simulink model "Telemetry_Test"  (Simulink 7.7)
settings: Solver=ode4  StartTime=0.0  StopTime=inf  FixedStep=sample_time_Vicon  RelTol=1e-3
InitFcn:
  | sample_time_Vicon = 0.004;
  | sample_time=0.02;
  | DeltaT = sample_time;
  | H0 = -0.36;
  | Kl = 1;
  | Omega_r =1.1; %1.3
settings Model: Creator=ttcl3  LastModifiedBy=Vicon
settings SolverCC: MaxConsecutiveMinStep=auto
settings OptimizationCC: EfficientMapNaN2IntZero=off
settings DebuggingCC: MultiTaskRateTransMsg=warning
settings HardwareCC: TargetIntDivRoundTo=Zero  TargetEndianess=LittleEndian  TargetHWDeviceType=MATLAB Host  ProdEqTarget=off
settings SFSimCC: SimParseCustomCode=off
settings CodeAppCC: MaxIdLength=128

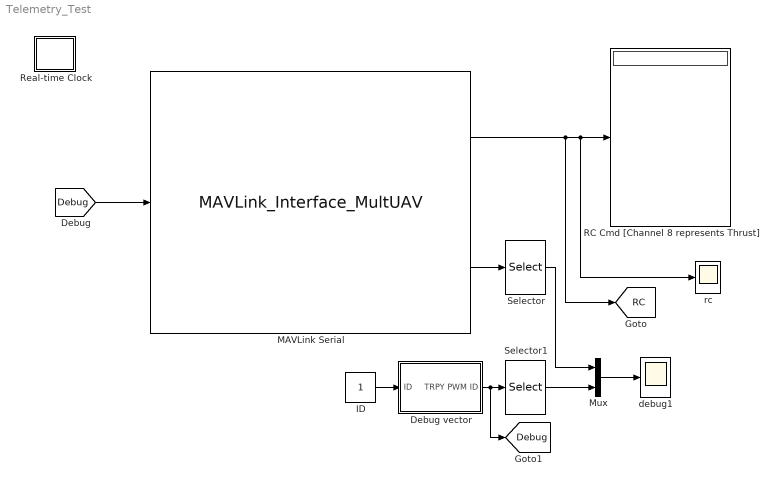
== system Telemetry_Test ==
  Debug vector : Subsystem
  ID : Constant
  MAVLink Serial : S-Function  FunctionName=MAVLink_Interface_MultUAV  Parameters=COM_Port,Baud_Rate,MSG_INPUT,MSG_OUTPUT  EnableBusSupport=off  mask{COM_Port='COM7', Baud_Rate=57600, ATTITUDE_OUT=on, RC_SCALED=on, Quad_1=off, Quad_2=off, Quad_3=off, Quad_4=off, Quad_5=off, Quad_6=off, Quad_7=on, Quad_8=off, Quad_9=off, Quad_10=off, Quad_11=off, Quad_12=off, Quad_13=off, Quad_14=off, Quad_15=off, Quad_16=off, Quad_17=off, Quad_18=off, Quad_19=off, Quad_20=off, Quad_21=off, Quad_22=off, Quad_23=off, Quad_24=off, Quad_25=off, Quad_26=off, Quad_27=off, Quad_28=off, Quad_29=off, Quad_30=off}
      mask prompts: COM_Port "COM Port"; Baud_Rate "Baud Rate"; ATTITUDE_OUT "ATTITUDE"; RC_SCALED "RC CHANNELS SCALED"; Quad_1 "Quad No 1"; Quad_2 "Quad No 2"; Quad_3 "Quad No 3"; Quad_4 "Quad No 4"; Quad_5 "Quad No 5"; Quad_6 "Quad No 6"; Quad_7 "Quad No 7"; Quad_8 "Quad No 8"; Quad_9 "Quad No 9"; Quad_10 "Quad No 10"; Quad_11 "Quad No 11"; Quad_12 "Quad No 12"; Quad_13 "Quad No 13"; Quad_14 "Quad No 14"; Quad_15 "Quad No 15"; Quad_16 "Quad No 16"; Quad_17 "Quad No 17"; Quad_18 "Quad No 18"; Quad_19 "Quad No 19"; Quad_20 "Quad No 20"; Quad_21 "Quad No 21"; Quad_22 "Quad No 22"; Quad_23 "Quad No 23"; Quad_24 "Quad No 24"; Quad_25 "Quad No 25"; Quad_26 "Quad No 26"; Quad_27 "Quad No 27"; Quad_28 "Quad No 28"; Quad_29 "Quad No 29"; Quad_30 "Quad No 30"
      mask init:
      | MSG_ID_NUM_INPUT = [uint8(196) uint8(197) uint8(198) uint8(199) uint8(200) uint8(201) uint8(202) uint8(203) uint8(204) uint8(205)
      |                     uint8(206) uint8(207) uint8(208) uint8(209) uint8(210) uint8(211) uint8(212) uint8(213) uint8(214) uint8(215)
      |                     uint8(216) uint8(217) uint8(218) uint8(219) uint8(220) uint8(221) uint8(222) uint8(223) uint8(224) uint8(225)];
      | MSG_ID_NAME_INPUT = [Quad_1 Quad_2 Quad_3 Quad_4 Quad_5 Quad_6 Quad_7 Quad_8 Quad_9 Quad_10
      |                      Quad_11 Quad_12 Quad_13 Quad_14 Quad_15 Quad_16 Quad_17 Quad_18 Quad_19 Quad_20
      |                      Quad_21 Quad_22 Quad_23 Quad_24 Quad_25 Quad_26 Quad_27 Quad_28 Quad_29 Quad_30];
      | 
      | MSG_ID_NUM_OUTPUT = [uint8(34) uint8(30)];
      | MSG_ID_NAME_OUTPUT = [RC_SCALED ATTITUDE_OUT ];
      | 
      | idx_input = find(MSG_ID_NAME_INPUT);
      | MSG_INPUT = MSG_ID_NUM_INPUT(idx_input);
      | 
      | idx_output = find(MSG_ID_NAME_OUTPUT);
      | MSG_OUTPUT = MSG_ID_NUM_OUTPUT(idx_output);
      mask TabNameString: Setting,Setting,Output Message,Output Message,Input Message,Input Message,Input Message,Input Message,Input Message,Input Message,Input Message,Input Message,Input Message,Input Message,Input Message,Input Message,Input Message,Input Message,Input Message,Input Message,Input Message,Input Message,Input Message,Input Message,Input Message,Input Message,Input Message,Input Message,Input Message,Input Message,Input Message,Input Message,Input Message,Input Message
      mask Display:
      | % Block image
      | image(imread('10-inch Quad Heat Map.png'));
      | 
      | %Label block
      | fprintf('MAVLink Serial\n%s\n%dbps', COM_Port,  Baud_Rate)
      | 
      | 
      | %Label input ports
      | 
      | in = 1;
      | if (Quad_1 == 1)
      |     port_label('input', in, 'Quad 1');
      |     in = in + 1;
      | end
      | if (Quad_2 == 1)
      |     port_label('input', in, 'Quad 2');
      |     in = in + 1;
      | end
      | 
      | if (Quad_3 == 1)
      |     port_label('input', in, 'Quad 3');
      |     in = in + 1;
      | end
      | 
      | if (Quad_4 == 1)
      |     port_label('input', in, 'Quad 4');
      |     in = in + 1;
      | end
      | 
      | if (Quad_5 == 1)
      |     port_label('input', in, 'Quad 5');
      |     in = in + 1;
      | end
      | 
      | if (Quad_6 == 1)
      |     port_label('input', in, 'Quad 6');
      |     in = in + 1;
      | end
      | 
      | if (Quad_7 == 1)
      |     port_label('input', in, 'Quad 7');
      |     in = in + 1;
      | end
      | 
      | if (Quad_8 == 1)
      |     port_label('input', in, 'Quad 8');
      |     in = in + 1;
      | end
      | 
      | if (Quad_9 == 1)
      |     port_label('input', in, 'Quad 9');
      |     in = in + 1;
      | end
      | 
      | if (Quad_10 == 1)
      |     port_label('input', in, 'Quad 10');
      |     in = in + 1;
      | end
      | 
      | if (Quad_11 == 1)
      |     port_label('input', in, 'Quad 11');
      |     in = in + 1;
      | end
      | 
      | if (Quad_12 == 1)
      |     port_label('input', in, 'Quad 12');
      |     in = in + 1;
      | end
      | 
      | if (Quad_13 == 1)
      |     port_label('input', in, 'Quad 13');
      |     in = in + 1;
      | end
      | 
      | if (Quad_14 == 1)
      |     port_label('input', in, 'Quad 14');
      |     in = in + 1;
      | end
      | 
      | if (Quad_15 == 1)
      |     port_label('input', in, 'Quad 15');
      |     in = in + 1;
      | end
      | 
      | if (Quad_16 == 1)
      |     port_label('input', in, 'Quad 16');
      |     in = in + 1;
      | end
      | 
      | if (Quad_17 == 1)
      |     port_label('input', in, 'Quad 17');
      |     in = in + 1;
      | end
      | 
      | if (Quad_18 == 1)
      |     port_label('input', in, 'Quad 18');
      |     in = in + 1;
      | end
      | 
      | 
      | if (Quad_19 == 1)
      |     port_label('input', in, 'Quad 19');
      |     in = in + 1;
      | end
      | 
      | if (Quad_20 == 1)
      |     port_label('input', in, 'Quad 20');
      |     in = in + 1;
      | end
      | 
      | if (Quad_21 == 1)
      |     port_label('input', in, 'Quad 21');
      |     in = in + 1;
      | end
      | 
      | if (Quad_22 == 1)
      |     port_label('input', in, 'Quad 22');
      |     in = in + 1;
      | end
      | 
      | if (Quad_23 == 1)
      |     port_label('input', in, 'Quad 23');
      |     in = in + 1;
      | end
      | 
      | if (Quad_24 == 1)
      |     port_label('input', in, 'Quad 24');
      |     in = in + 1;
      | end
      | 
      | if (Quad_25 == 1)
      |     port_label('input', in, 'Quad 25');
      |     in = in + 1;
      | end
      | 
      | if (Quad_26 == 1)
      |     port_label('input', in, 'Quad 26');
      |     in = in + 1;
      | end
      | 
      | if (Quad_27 == 1)
      |     port_label('input', in, 'Quad 27');
      |     in = in + 1;
      | end
      | 
      | if (Quad_28 == 1)
      |     port_label('input', in, 'Quad 28');
      |     in = in + 1;
      | end
      | 
      | if (Quad_29 == 1)
      |     port_label('input', in, 'Quad 29');
      |     in = in + 1;
      | end
      | 
      | if (Quad_30 == 1)
      |     port_label('input', in, 'Quad 30');
      |     in = in + 1;
      | end
      | %Label output ports
      | 
      | out = 1;
      | if (RC_SCALED == 1)
      |     port_label('output', out, 'RC CMD');
      |     out = out + 1;
      | end
      | 
      | if (ATTITUDE_OUT == 1)
      |     port_label('output', out, 'DEBUG');
      |     out = out + 1;
      | end
  Mux : Mux  Inputs=2
  RC Cmd [Channel 8 represents Thrust] : Display
  Real-time Clock : Subsystem  mask(Real-time Clock){sample_time=sample_time, tolerance=0.03}
      mask prompts: sample_time "Synchronize with real-time every n seconds:"; tolerance "Real-time warning tolerance (seconds):"
      mask help: Real-time Synchronization Block
      mask Help: This block synchronizes simulation time with the PC real-time clock or UNIX system clock. The first dialog entry is the period at which the clock is checked to insure real-time synchronization. The second dialog entry is the number of seconds that the simulation time must be within real-time before a warning is printed.
      mask Display: plot(0,0,100,100,[40,60,60,54,54,64,69,76,82,77,81,83,83,81,78,74,70,64,57,49,41,35,32,30,30,31,34,40,47,47,40,40],[90,90,85,85,80,79,76,87,80,70,64,57,49,41,33,28,24,22,21,23,25,31,37,46,56,65,73,78,80,85,85,90],[69,53,53],[64,50,73])
  Selector : Selector  InputPortWidth=6  IndexOptions=Index vector (dialog)  Indices=[3]  OutputSizes=1
  Selector1 : Selector  InputPortWidth=6  IndexOptions=Index vector (dialog)  Indices=1  OutputSizes=1
  debug1 : Scope
      settings: TimeRange=10  YMin=-1  YMax=1  SaveName=ScopeData2
  rc : Scope
      settings: TimeRange=10  YMin=-1  YMax=0.05
  tag scope: Debug=global, RC=global
  wires:
  MAVLink Serial/1 -> [RC], RC Cmd [Channel 8 represents Thrust]/1, rc/1
  Mux/1 -> debug1/1
  Debug vector/1(TRPY PWM ID) -> Selector1/1, [Debug]
  ID/1 -> Debug vector/1(ID)
  Selector/1 -> Mux/1
  Selector1/1 -> Mux/2
  MAVLink Serial/2 -> Selector/1
  [Debug] -> MAVLink Serial/1

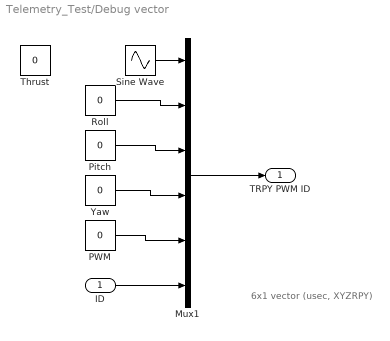
== system Telemetry_Test/Debug vector ==
  note: 6x1 vector (usec, XYZRPY)
  ID : Inport
  Mux1 : Mux  Inputs=6
  PWM : Constant  Value=0
  Pitch : Constant  Value=0
  Roll : Constant  Value=0
  Sine Wave : Sin  SampleTime=0
  Thrust : Constant  Value=0
  Yaw : Constant  Value=0
  TRPY PWM ID : Outport
  wires:
  Mux1/1 -> TRPY PWM ID/1
  Roll/1 -> Mux1/2
  Pitch/1 -> Mux1/3
  Yaw/1 -> Mux1/4
  PWM/1 -> Mux1/5
  ID/1 -> Mux1/6
  Sine Wave/1 -> Mux1/1

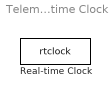
== system Telemetry_Test/Real-time Clock ==
  Real-time Clock : S-Function  FunctionName=rtclock  Parameters=sample_time, tolerance  EnableBusSupport=off
